simulink model "plant"  (R2015a)
settings: Solver=FixedStepDiscrete  StartTime=0.0  StopTime=10.0  RelTol=1e-3
undefined symbols (not defined in the file or in its folder): A, B, C
settings Model: Creator=alunos  LastModifiedBy=Hugo
settings DataIOCC: LimitDataPoints=off

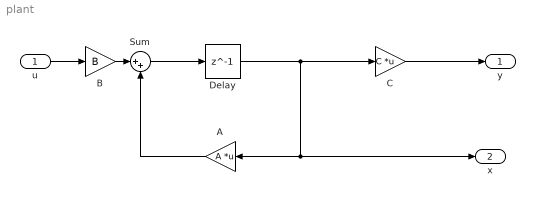
== system plant ==
  u : Inport
  A : Gain  Gain=A  Multiplication=Matrix(K*u)
  B : Gain  Gain=B
  C : Gain  Gain=C  Multiplication=Matrix(K*u)
  Delay : Delay  DelayLength=1  InitialCondition=[0;0;0;0]
  Sum : Sum  Inputs=|++
  y : Outport
  x : Outport  Port=2
  wires:
  C/1 -> y/1
  B/1 -> Sum/1
  Sum/1 -> Delay/1
  A/1 -> Sum/2
  u/1 -> B/1
  Delay/1 -> x/1, A/1, C/1
